simulink model "tank_reactor_no_error_dyn"  (R2020a)
settings: Solver=FixedStepAuto  StartTime=0.0  StopTime=options.T_train  FixedStep=options.dt  RelTol=1e-3
PreLoadFcn:
  | load PIDGainSchedExample.mat
model workspace (MAT data in the model file):
  op_snapshot1 : handle (value not decoded)
undefined symbols (not defined in the file or in its folder): C, Controllers, D, I, N, options, P, sigbuilder_block
libraries: neural x132, simulink x2, simulink_need_slupdate x1
(part 2 of 6)

== system tank_reactor_no_error_dyn/NN/Layer 1/Delays 1 ==
  "p{1}" : Inport  PortDimensions=8
      mask Display: e = 0.06;c1 = [120 230 180]/255;c2 = ([120 230 180]+0)/(256+128);c3 = ([120 230 180]+128)/(256+128);patch([0 1 1 0],[0 0 1 1],c1);patch([0 1 1 1-e 1-e 0+e],[0 0 1 1-e 0+e 0+e],c2);patch([0 0 1 1-e 0+e 0+e],[0 1 1 1-e 1-e 0+e],c3);plot([0 1 1 0 0],[0 0 1 1 0]);
  mux : Mux  Inputs=1
      mask Display: e = 0.06;c1 = [120 150 230]/255;c2 = ([120 150 230]+0)/383;c3 = ([120 150 230]+128)/383;patch([0 1 1 0],[0 0 1 1],c1);patch([0 1 1 1-e 1-e 0+e],[0 0 1 1-e 0+e 0+e],c2);patch([0 0 1 1-e 0+e 0+e],[0 1 1 1-e 1-e 0+e],c3);plot([0 1 1 0 0],[0 0 1 1 0]);disp('Mux')
  "pd{1,1}" : Outport
      mask Display: e = 0.06;c1 = [120 230 180]/255;c2 = ([120 230 180]+0)/(256+128);c3 = ([120 230 180]+128)/(256+128);patch([0 1 1 0],[0 0 1 1],c1);patch([0 1 1 1-e 1-e 0+e],[0 0 1 1-e 0+e 0+e],c2);patch([0 0 1 1-e 0+e 0+e],[0 1 1 1-e 1-e 0+e],c3);plot([0 1 1 0 0],[0 0 1 1 0]);
  wires:
  "p{1}"/1 -> mux/1
  mux/1 -> "pd{1,1}"/1

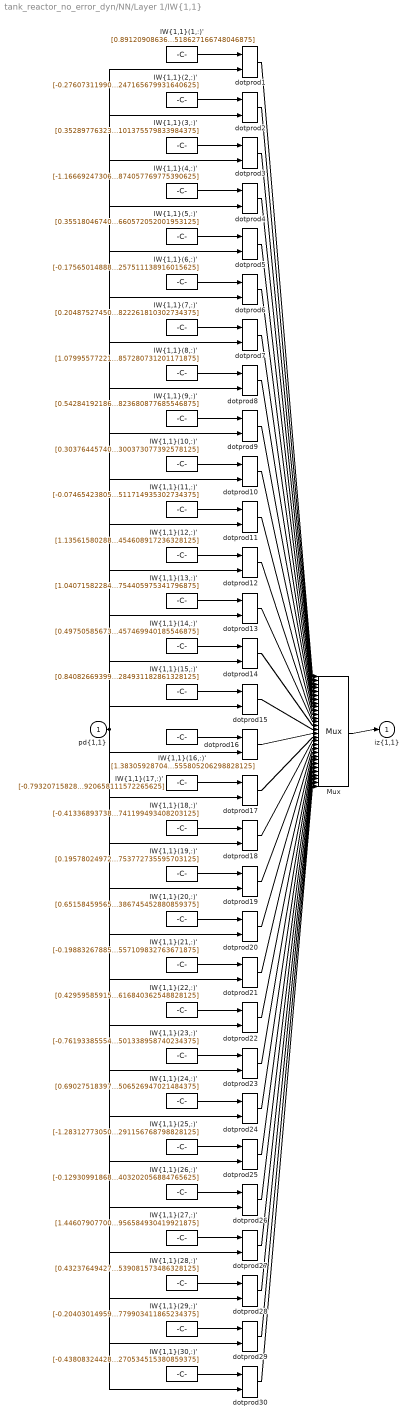
== system tank_reactor_no_error_dyn/NN/Layer 1/IW{1,1} ==
  "pd{1,1}" : Inport  PortDimensions=8
      mask Display: e = 0.06;c1 = [120 230 180]/255;c2 = ([120 230 180]+0)/(256+128);c3 = ([120 230 180]+128)/(256+128);patch([0 1 1 0],[0 0 1 1],c1);patch([0 1 1 1-e 1-e 0+e],[0 0 1 1-e 0+e 0+e],c2);patch([0 0 1 1-e 0+e 0+e],[0 1 1 1-e 1-e 0+e],c3);plot([0 1 1 0 0],[0 0 1 1 0]);
  "IW{1,1}(1,:)'" : Constant  Value=[0.891209086360823743433456911589019000530242919921875;-0.000910908649453586708073793420936681286548264324665069580078125;0.16926229689930305521983200378599576652050018310546875;0.0961010344390704762673749428358860313892364501953125;-0.71802013876261872038497813264257274568080902099609375;-1.2927237305927830046670123920193873345851898193359375;0.90818838200151918993441313432413153350353240966796875;0.427072169502839382726477879259618930518627166748046875]
      mask Display: e = 0.06;c1 = [120 150 230]/255;c2 = ([120 150 230]+0)/383;c3 = ([120 150 230]+128)/383;patch([0 1 1 0],[0 0 1 1],c1);patch([0 1 1 1-e 1-e 0+e],[0 0 1 1-e 0+e 0+e],c2);patch([0 0 1 1-e 0+e 0+e],[0 1 1 1-e 1-e 0+e],c3);plot([0 1 1 0 0],[0 0 1 1 0]);disp('Weights');
  "IW{1,1}(10,:)'" : Constant  Value=[0.303764457407485977125105591767351143062114715576171875;-1.996551308659621160046526711084879934787750244140625;1.2595053737837555996037508521112613379955291748046875;-1.02115406267071673340751658543013036251068115234375;2.473413894732976014978476086980663239955902099609375;-0.7761438730779877115395493092364631593227386474609375;-0.71002775511161775323643041701870970427989959716796875;0.1135875630970302474498367928390507586300373077392578125]
      mask Display: e = 0.06;c1 = [120 150 230]/255;c2 = ([120 150 230]+0)/383;c3 = ([120 150 230]+128)/383;patch([0 1 1 0],[0 0 1 1],c1);patch([0 1 1 1-e 1-e 0+e],[0 0 1 1-e 0+e 0+e],c2);patch([0 0 1 1-e 0+e 0+e],[0 1 1 1-e 1-e 0+e],c3);plot([0 1 1 0 0],[0 0 1 1 0]);disp('Weights');
  "IW{1,1}(11,:)'" : Constant  Value=[-0.07465423805538810853033027115088771097362041473388671875;1.8872792622725416133988574074464850127696990966796875;-0.28367390430513361732067778575583361089229583740234375;-0.60649854229973543251475120996474288403987884521484375;-1.1760495898640888068342746919370256364345550537109375;2.003426546042650802093021411565132439136505126953125;0.51689646511757303404266394863952882587909698486328125;-0.92364179088715070431447884402587078511714935302734375]
      mask Display: e = 0.06;c1 = [120 150 230]/255;c2 = ([120 150 230]+0)/383;c3 = ([120 150 230]+128)/383;patch([0 1 1 0],[0 0 1 1],c1);patch([0 1 1 1-e 1-e 0+e],[0 0 1 1-e 0+e 0+e],c2);patch([0 0 1 1-e 0+e 0+e],[0 1 1 1-e 1-e 0+e],c3);plot([0 1 1 0 0],[0 0 1 1 0]);disp('Weights');
  "IW{1,1}(12,:)'" : Constant  Value=[1.1356158028888374555975815383135341107845306396484375;-0.8606555624373211088595780893228948116302490234375;1.062201621871125656326739772339351475238800048828125;0.385334575489824970873087295331060886383056640625;-1.0206910368916128906136009391047991812229156494140625;-0.76634897790539968642775647822418250143527984619140625;0.71194817031437462873100230353884398937225341796875;-0.684976270533752984448483402957208454608917236328125]
      mask Display: e = 0.06;c1 = [120 150 230]/255;c2 = ([120 150 230]+0)/383;c3 = ([120 150 230]+128)/383;patch([0 1 1 0],[0 0 1 1],c1);patch([0 1 1 1-e 1-e 0+e],[0 0 1 1-e 0+e 0+e],c2);patch([0 0 1 1-e 0+e 0+e],[0 1 1 1-e 1-e 0+e],c3);plot([0 1 1 0 0],[0 0 1 1 0]);disp('Weights');
  "IW{1,1}(13,:)'" : Constant  Value=[1.040715822845224902692962132277898490428924560546875;-1.20594832363064963232091031386516988277435302734375;-0.72554525921453905112912252661772072315216064453125;-0.58377306366834436079926717866328544914722442626953125;0.85741126153984448254874450867646373808383941650390625;-0.71285015732533185683905685436911880970001220703125;-0.294932600157362390103088500836747698485851287841796875;-0.392736442125421081339453621694701723754405975341796875]
      mask Display: e = 0.06;c1 = [120 150 230]/255;c2 = ([120 150 230]+0)/383;c3 = ([120 150 230]+128)/383;patch([0 1 1 0],[0 0 1 1],c1);patch([0 1 1 1-e 1-e 0+e],[0 0 1 1-e 0+e 0+e],c2);patch([0 0 1 1-e 0+e 0+e],[0 1 1 1-e 1-e 0+e],c3);plot([0 1 1 0 0],[0 0 1 1 0]);disp('Weights');
  "IW{1,1}(14,:)'" : Constant  Value=[0.49750585673530112185147800119011662900447845458984375;-0.54863714662622420359383568211342208087444305419921875;0.98098386380823310304322149022482335567474365234375;0.0235222284456758322368497005072640604339540004730224609375;-0.2518678635057340908787182343075983226299285888671875;0.87089778090608327421051626515691168606281280517578125;-0.84448838533145298423931990328128449618816375732421875;0.64158694309444352921190102279069833457469940185546875]
      mask Display: e = 0.06;c1 = [120 150 230]/255;c2 = ([120 150 230]+0)/383;c3 = ([120 150 230]+128)/383;patch([0 1 1 0],[0 0 1 1],c1);patch([0 1 1 1-e 1-e 0+e],[0 0 1 1-e 0+e 0+e],c2);patch([0 0 1 1-e 0+e 0+e],[0 1 1 1-e 1-e 0+e],c3);plot([0 1 1 0 0],[0 0 1 1 0]);disp('Weights');
  "IW{1,1}(15,:)'" : Constant  Value=[0.8408266939989401667077117963344790041446685791015625;-0.6803304612663236827785340210539288818836212158203125;0.909265244574289255297117051668465137481689453125;-1.9435766040642281637929045245982706546783447265625;-0.57838745834684257562940956631791777908802032470703125;0.339153364989726535672076579430722631514072418212890625;0.66688594346699681114642999091302044689655303955078125;-0.98381930870071443440139091762830503284931182861328125]
      mask Display: e = 0.06;c1 = [120 150 230]/255;c2 = ([120 150 230]+0)/383;c3 = ([120 150 230]+128)/383;patch([0 1 1 0],[0 0 1 1],c1);patch([0 1 1 1-e 1-e 0+e],[0 0 1 1-e 0+e 0+e],c2);patch([0 0 1 1-e 0+e 0+e],[0 1 1 1-e 1-e 0+e],c3);plot([0 1 1 0 0],[0 0 1 1 0]);disp('Weights');
  "IW{1,1}(16,:)'" : Constant  Value=[1.3830592870458413568002242755028419196605682373046875;1.0887774896799757851084677895414642989635467529296875;1.271992703112938105647344855242408812046051025390625;-1.1783294637027565965325948127429001033306121826171875;1.1046083450996917463271529413759708404541015625;-0.313172955783324102885245565630611963570117950439453125;-0.708707743855683691691638159682042896747589111328125;0.18575113039401813797013574003358371555805206298828125]
      mask Display: e = 0.06;c1 = [120 150 230]/255;c2 = ([120 150 230]+0)/383;c3 = ([120 150 230]+128)/383;patch([0 1 1 0],[0 0 1 1],c1);patch([0 1 1 1-e 1-e 0+e],[0 0 1 1-e 0+e 0+e],c2);patch([0 0 1 1-e 0+e 0+e],[0 1 1 1-e 1-e 0+e],c3);plot([0 1 1 0 0],[0 0 1 1 0]);disp('Weights');
  "IW{1,1}(17,:)'" : Constant  Value=[-0.7932071582841186963008794919005595147609710693359375;-0.69262888914015141583746526521281339228153228759765625;1.1347110976433001372498665659804828464984893798828125;0.471156780921254736416159403233905322849750518798828125;1.391933236785583449801606548135168850421905517578125;0.76600648986104047377665438034455291926860809326171875;1.4849938450647390819625570657080970704555511474609375;-0.12300708250844562263726089668125496245920658111572265625]
      mask Display: e = 0.06;c1 = [120 150 230]/255;c2 = ([120 150 230]+0)/383;c3 = ([120 150 230]+128)/383;patch([0 1 1 0],[0 0 1 1],c1);patch([0 1 1 1-e 1-e 0+e],[0 0 1 1-e 0+e 0+e],c2);patch([0 0 1 1-e 0+e 0+e],[0 1 1 1-e 1-e 0+e],c3);plot([0 1 1 0 0],[0 0 1 1 0]);disp('Weights');
  "IW{1,1}(18,:)'" : Constant  Value=[-0.41336893738068003489871671263244934380054473876953125;0.34606769462915309976125399771262891590595245361328125;0.6930097657111240483374103860114701092243194580078125;-0.0245843145830253462236214545555412769317626953125;0.0774614107242942162567800323813571594655513763427734375;-1.420788434284315115974095533601939678192138671875;0.7440334973332751733465784127474762499332427978515625;-0.67774743533416892393717034792643971741199493408203125]
      mask Display: e = 0.06;c1 = [120 150 230]/255;c2 = ([120 150 230]+0)/383;c3 = ([120 150 230]+128)/383;patch([0 1 1 0],[0 0 1 1],c1);patch([0 1 1 1-e 1-e 0+e],[0 0 1 1-e 0+e 0+e],c2);patch([0 0 1 1-e 0+e 0+e],[0 1 1 1-e 1-e 0+e],c3);plot([0 1 1 0 0],[0 0 1 1 0]);disp('Weights');
  "IW{1,1}(19,:)'" : Constant  Value=[0.195780249723398913630489914794452488422393798828125;1.5706960428444365351907663352903909981250762939453125;-0.022910753267789296661050002512638457119464874267578125;0.07656576370324440217185468782190582714974880218505859375;-1.8746061388155847993175484589301049709320068359375;1.197653751465737936854338840930722653865814208984375;1.678192708089004003824129540589638054370880126953125;-0.257162313468550618456021084057283587753772735595703125]
      mask Display: e = 0.06;c1 = [120 150 230]/255;c2 = ([120 150 230]+0)/383;c3 = ([120 150 230]+128)/383;patch([0 1 1 0],[0 0 1 1],c1);patch([0 1 1 1-e 1-e 0+e],[0 0 1 1-e 0+e 0+e],c2);patch([0 0 1 1-e 0+e 0+e],[0 1 1 1-e 1-e 0+e],c3);plot([0 1 1 0 0],[0 0 1 1 0]);disp('Weights');
  "IW{1,1}(2,:)'" : Constant  Value=[-0.27607311990221428121827784707420505583286285400390625;3.19576707068835474956358666531741619110107421875;-1.0428488373978215264514801674522459506988525390625;0.33427289240207846976460359655902720987796783447265625;-0.786125397896479061188301784568466246128082275390625;-0.062361390428662490104105842192439013160765171051025390625;1.2065016053652370953130912312190048396587371826171875;-0.394134012811458378511275668643065728247165679931640625]
      mask Display: e = 0.06;c1 = [120 150 230]/255;c2 = ([120 150 230]+0)/383;c3 = ([120 150 230]+128)/383;patch([0 1 1 0],[0 0 1 1],c1);patch([0 1 1 1-e 1-e 0+e],[0 0 1 1-e 0+e 0+e],c2);patch([0 0 1 1-e 0+e 0+e],[0 1 1 1-e 1-e 0+e],c3);plot([0 1 1 0 0],[0 0 1 1 0]);disp('Weights');
  "IW{1,1}(20,:)'" : Constant  Value=[0.65158459565695447945898877151194028556346893310546875;-0.54696539429589241532170262871659360826015472412109375;-0.54826498940842782747751016358961351215839385986328125;-0.65072656451431776236660198264871723949909210205078125;0.0708601621656460844977942770128720439970493316650390625;-1.6283005755519279755816342003527097404003143310546875;0.77614797039212113372030898972298018634319305419921875;1.307748898949637972322079804143868386745452880859375]
      mask Display: e = 0.06;c1 = [120 150 230]/255;c2 = ([120 150 230]+0)/383;c3 = ([120 150 230]+128)/383;patch([0 1 1 0],[0 0 1 1],c1);patch([0 1 1 1-e 1-e 0+e],[0 0 1 1-e 0+e 0+e],c2);patch([0 0 1 1-e 0+e 0+e],[0 1 1 1-e 1-e 0+e],c3);plot([0 1 1 0 0],[0 0 1 1 0]);disp('Weights');
  "IW{1,1}(21,:)'" : Constant  Value=[-0.198832678858577527325479650244233198463916778564453125;-1.5667262584966288319066052281414158642292022705078125;0.60294794988579614170021159225143492221832275390625;1.0351174578473163467862150355358608067035675048828125;0.57511724013551501766272622262476943433284759521484375;-1.9983892082063359207921848792466334998607635498046875;1.087121479066192275553248691721819341182708740234375;-0.085864453590817901851295346205006353557109832763671875]
      mask Display: e = 0.06;c1 = [120 150 230]/255;c2 = ([120 150 230]+0)/383;c3 = ([120 150 230]+128)/383;patch([0 1 1 0],[0 0 1 1],c1);patch([0 1 1 1-e 1-e 0+e],[0 0 1 1-e 0+e 0+e],c2);patch([0 0 1 1-e 0+e 0+e],[0 1 1 1-e 1-e 0+e],c3);plot([0 1 1 0 0],[0 0 1 1 0]);disp('Weights');
  "IW{1,1}(22,:)'" : Constant  Value=[0.42959585915928055754875458660535514354705810546875;1.608771338683758767018616708810441195964813232421875;-1.0989417017832732170745657640509307384490966796875;0.371220710965206202036625882101361639797687530517578125;-0.2473361319530964774759951296800863929092884063720703125;-0.69784269808488785802325082840980030596256256103515625;-0.27799942923109954850957592498161830008029937744140625;0.43439637348526460858266773357172496616840362548828125]
      mask Display: e = 0.06;c1 = [120 150 230]/255;c2 = ([120 150 230]+0)/383;c3 = ([120 150 230]+128)/383;patch([0 1 1 0],[0 0 1 1],c1);patch([0 1 1 1-e 1-e 0+e],[0 0 1 1-e 0+e 0+e],c2);patch([0 0 1 1-e 0+e 0+e],[0 1 1 1-e 1-e 0+e],c3);plot([0 1 1 0 0],[0 0 1 1 0]);disp('Weights');
  "IW{1,1}(23,:)'" : Constant  Value=[-0.76193385554215853350257248166599310934543609619140625;-1.168991754040985764362403642735444009304046630859375;1.16775652995662237998431010055355727672576904296875;-0.8596786858297369438020041343406774103641510009765625;1.1885630047108375340059183145058341324329376220703125;0.6353358394109431817042832335573621094226837158203125;0.73915724568664809002171978136175312101840972900390625;0.087989459536861269750573910641833208501338958740234375]
      mask Display: e = 0.06;c1 = [120 150 230]/255;c2 = ([120 150 230]+0)/383;c3 = ([120 150 230]+128)/383;patch([0 1 1 0],[0 0 1 1],c1);patch([0 1 1 1-e 1-e 0+e],[0 0 1 1-e 0+e 0+e],c2);patch([0 0 1 1-e 0+e 0+e],[0 1 1 1-e 1-e 0+e],c3);plot([0 1 1 0 0],[0 0 1 1 0]);disp('Weights');
  "IW{1,1}(24,:)'" : Constant  Value=[0.6902751839763094920954245026223361492156982421875;-1.1906714422756998761343538717483170330524444580078125;0.82139232284612184731287243266706354916095733642578125;-1.1361593673824572636732455066521652042865753173828125;-0.09408198905645491494365018070311634801328182220458984375;0.379573069658633299727767962394864298403263092041015625;-0.2275798022518404628566912606402183882892131805419921875;0.76388497817848433069087832336663268506526947021484375]
      mask Display: e = 0.06;c1 = [120 150 230]/255;c2 = ([120 150 230]+0)/383;c3 = ([120 150 230]+128)/383;patch([0 1 1 0],[0 0 1 1],c1);patch([0 1 1 1-e 1-e 0+e],[0 0 1 1-e 0+e 0+e],c2);patch([0 0 1 1-e 0+e 0+e],[0 1 1 1-e 1-e 0+e],c3);plot([0 1 1 0 0],[0 0 1 1 0]);disp('Weights');
  "IW{1,1}(25,:)'" : Constant  Value=[-1.283127730500394303447819766006432473659515380859375;-0.82493970737477162469275526746059767901897430419921875;-0.324102141434564117172811847922275774180889129638671875;-0.28127820987730556279160509802750311791896820068359375;-1.0514780139675818926292549804202280938625335693359375;0.7115020200138741923723273430368863046169281005859375;-0.427400400411290071200909324034000746905803680419921875;0.75331051910044621866546776800532825291156768798828125]
      mask Display: e = 0.06;c1 = [120 150 230]/255;c2 = ([120 150 230]+0)/383;c3 = ([120 150 230]+128)/383;patch([0 1 1 0],[0 0 1 1],c1);patch([0 1 1 1-e 1-e 0+e],[0 0 1 1-e 0+e 0+e],c2);patch([0 0 1 1-e 0+e 0+e],[0 1 1 1-e 1-e 0+e],c3);plot([0 1 1 0 0],[0 0 1 1 0]);disp('Weights');
  "IW{1,1}(26,:)'" : Constant  Value=[-0.1293099186855697357856342932791449129581451416015625;2.312536055211477314941248550894670188426971435546875;-1.886850622227131513142239782609976828098297119140625;0.6923975867468554756811727202148176729679107666015625;-0.51896714360574291990957362941117025911808013916015625;-1.232082621271291866804631354170851409435272216796875;0.338074964824850721090143679248285479843616485595703125;-0.17734705034791053979148500729934312403202056884765625]
      mask Display: e = 0.06;c1 = [120 150 230]/255;c2 = ([120 150 230]+0)/383;c3 = ([120 150 230]+128)/383;patch([0 1 1 0],[0 0 1 1],c1);patch([0 1 1 1-e 1-e 0+e],[0 0 1 1-e 0+e 0+e],c2);patch([0 0 1 1-e 0+e 0+e],[0 1 1 1-e 1-e 0+e],c3);plot([0 1 1 0 0],[0 0 1 1 0]);disp('Weights');
  "IW{1,1}(27,:)'" : Constant  Value=[1.4460790770033928875903939115232788026332855224609375;-1.174753989253496389011388600920327007770538330078125;-0.903663094360668051052698501734994351863861083984375;1.2089315703201017893064772579236887395381927490234375;-1.5344822755058282748308329246356151998043060302734375;-1.2575764011052263935397377281333319842815399169921875;0.27661093956695115281263497308827936649322509765625;-0.309828444908113009859107478405348956584930419921875]
      mask Display: e = 0.06;c1 = [120 150 230]/255;c2 = ([120 150 230]+0)/383;c3 = ([120 150 230]+128)/383;patch([0 1 1 0],[0 0 1 1],c1);patch([0 1 1 1-e 1-e 0+e],[0 0 1 1-e 0+e 0+e],c2);patch([0 0 1 1-e 0+e 0+e],[0 1 1 1-e 1-e 0+e],c3);plot([0 1 1 0 0],[0 0 1 1 0]);disp('Weights');
  "IW{1,1}(28,:)'" : Constant  Value=[0.43237649427624680331661011223332025110721588134765625;0.248579972511031643822576597813167609274387359619140625;0.12073941905091711834785428436589427292346954345703125;-0.247775766713915046590699375883559696376323699951171875;-1.41605228232816227063040059874765574932098388671875;-0.250253560258686669204308827829663641750812530517578125;-0.9320172798745807174469746314571239054203033447265625;0.12770737221969341579352885673870332539081573486328125]
      mask Display: e = 0.06;c1 = [120 150 230]/255;c2 = ([120 150 230]+0)/383;c3 = ([120 150 230]+128)/383;patch([0 1 1 0],[0 0 1 1],c1);patch([0 1 1 1-e 1-e 0+e],[0 0 1 1-e 0+e 0+e],c2);patch([0 0 1 1-e 0+e 0+e],[0 1 1 1-e 1-e 0+e],c3);plot([0 1 1 0 0],[0 0 1 1 0]);disp('Weights');
  "IW{1,1}(29,:)'" : Constant  Value=[-0.20403014959684029339115340917487628757953643798828125;-1.2552046966677392614286645766696892678737640380859375;0.422075048629639237862676282020402140915393829345703125;0.457051193739799688220415418982156552374362945556640625;0.813647240052294051793069229461252689361572265625;0.94800113640993155517122659148299135267734527587890625;0.369592747067476079525505383571726270020008087158203125;-1.1506192330556908043348585124476812779903411865234375]
      mask Display: e = 0.06;c1 = [120 150 230]/255;c2 = ([120 150 230]+0)/383;c3 = ([120 150 230]+128)/383;patch([0 1 1 0],[0 0 1 1],c1);patch([0 1 1 1-e 1-e 0+e],[0 0 1 1-e 0+e 0+e],c2);patch([0 0 1 1-e 0+e 0+e],[0 1 1 1-e 1-e 0+e],c3);plot([0 1 1 0 0],[0 0 1 1 0]);disp('Weights');
  "IW{1,1}(3,:)'" : Constant  Value=[0.3528977632348235804471414667204953730106353759765625;0.1308640941319542394527530859704711474478244781494140625;-1.2444579430620941185026140374247916042804718017578125;0.83918272680140393315895153136807493865489959716796875;0.68037558300890565998741976727615110576152801513671875;-0.7022060286452938004941870531183667480945587158203125;-1.100538571020759359697649415466003119945526123046875;-0.6665379620285223349895886713056825101375579833984375]
      mask Display: e = 0.06;c1 = [120 150 230]/255;c2 = ([120 150 230]+0)/383;c3 = ([120 150 230]+128)/383;patch([0 1 1 0],[0 0 1 1],c1);patch([0 1 1 1-e 1-e 0+e],[0 0 1 1-e 0+e 0+e],c2);patch([0 0 1 1-e 0+e 0+e],[0 1 1 1-e 1-e 0+e],c3);plot([0 1 1 0 0],[0 0 1 1 0]);disp('Weights');
  "IW{1,1}(30,:)'" : Constant  Value=[-0.43808324428765110791772485754336230456829071044921875;0.41444371322705408910991309312521480023860931396484375;0.71121513137011527216913009397103451192378997802734375;-0.027277229924096473012706809413430164568126201629638671875;-1.37267882779404803983425154001452028751373291015625;-0.42987169918532674994793296718853525817394256591796875;-1.211486810975065164797115357941947877407073974609375;-0.6761643548908080614268101271591149270534515380859375]
      mask Display: e = 0.06;c1 = [120 150 230]/255;c2 = ([120 150 230]+0)/383;c3 = ([120 150 230]+128)/383;patch([0 1 1 0],[0 0 1 1],c1);patch([0 1 1 1-e 1-e 0+e],[0 0 1 1-e 0+e 0+e],c2);patch([0 0 1 1-e 0+e 0+e],[0 1 1 1-e 1-e 0+e],c3);plot([0 1 1 0 0],[0 0 1 1 0]);disp('Weights');
  "IW{1,1}(4,:)'" : Constant  Value=[-1.16669247306179446610485683777369558811187744140625;1.313151888737838834941840104875154793262481689453125;0.11554526367606703096679865439000423066318035125732421875;0.290758769956429963254862514077103696763515472412109375;-1.21604121550441401922171280602924525737762451171875;-0.34010080794086217093052937343600206077098846435546875;-0.1405823754041759243715858929135720245540142059326171875;0.1962377911275405839575114441686309874057769775390625]
      mask Display: e = 0.06;c1 = [120 150 230]/255;c2 = ([120 150 230]+0)/383;c3 = ([120 150 230]+128)/383;patch([0 1 1 0],[0 0 1 1],c1);patch([0 1 1 1-e 1-e 0+e],[0 0 1 1-e 0+e 0+e],c2);patch([0 0 1 1-e 0+e 0+e],[0 1 1 1-e 1-e 0+e],c3);plot([0 1 1 0 0],[0 0 1 1 0]);disp('Weights');
  "IW{1,1}(5,:)'" : Constant  Value=[0.355180467400776411768248408407089300453662872314453125;-1.1446138133397381064781939130625687539577484130859375;1.2998503170540998130633170148939825594425201416015625;-0.13732972862548187276132694023544900119304656982421875;0.88362338224945358167161657547694630920886993408203125;0.87567478655001151910397538813413120806217193603515625;-0.30563340366142954795947161983349360525608062744140625;-0.33053391115797670085640902470913715660572052001953125]
      mask Display: e = 0.06;c1 = [120 150 230]/255;c2 = ([120 150 230]+0)/383;c3 = ([120 150 230]+128)/383;patch([0 1 1 0],[0 0 1 1],c1);patch([0 1 1 1-e 1-e 0+e],[0 0 1 1-e 0+e 0+e],c2);patch([0 0 1 1-e 0+e 0+e],[0 1 1 1-e 1-e 0+e],c3);plot([0 1 1 0 0],[0 0 1 1 0]);disp('Weights');
  "IW{1,1}(6,:)'" : Constant  Value=[-0.1756501488876137939687538391808629967272281646728515625;1.4205293258788682653204205053043551743030548095703125;-0.300940034305634929179262826437479816377162933349609375;-0.1907224346195115216584525796861271373927593231201171875;-0.9385913103776528654265121076605282723903656005859375;-0.982602586260352683922292271745391190052032470703125;0.523715138108350242163169241393916308879852294921875;-0.447275069227227872747931769481510855257511138916015625]
      mask Display: e = 0.06;c1 = [120 150 230]/255;c2 = ([120 150 230]+0)/383;c3 = ([120 150 230]+128)/383;patch([0 1 1 0],[0 0 1 1],c1);patch([0 1 1 1-e 1-e 0+e],[0 0 1 1-e 0+e 0+e],c2);patch([0 0 1 1-e 0+e 0+e],[0 1 1 1-e 1-e 0+e],c3);plot([0 1 1 0 0],[0 0 1 1 0]);disp('Weights');
  "IW{1,1}(7,:)'" : Constant  Value=[0.2048752745045113454747109926756820641458034515380859375;1.3468461456425815381265920223086141049861907958984375;0.0036662755142019376290718479793895312468521296977996826171875;-0.5200031024826061720744974081753753125667572021484375;-1.6760754682220049271990092165651731193065643310546875;0.57178614216200951414492692492785863578319549560546875;0.7277091077803354846054162408108823001384735107421875;0.1111911977520590733004013372919871471822261810302734375]
      mask Display: e = 0.06;c1 = [120 150 230]/255;c2 = ([120 150 230]+0)/383;c3 = ([120 150 230]+128)/383;patch([0 1 1 0],[0 0 1 1],c1);patch([0 1 1 1-e 1-e 0+e],[0 0 1 1-e 0+e 0+e],c2);patch([0 0 1 1-e 0+e 0+e],[0 1 1 1-e 1-e 0+e],c3);plot([0 1 1 0 0],[0 0 1 1 0]);disp('Weights');
  "IW{1,1}(8,:)'" : Constant  Value=[1.0799557722149959460011814371682703495025634765625;-0.584193546292407717146488721482455730438232421875;-0.419015090910249465849801708827726542949676513671875;0.455745228535148483306471689502359367907047271728515625;-0.97753771333968086931776042547426186501979827880859375;0.475936941338956975844354246873990632593631744384765625;0.62248671937497668249505977655644528567790985107421875;-1.2675430185230183166567030639271251857280731201171875]
      mask Display: e = 0.06;c1 = [120 150 230]/255;c2 = ([120 150 230]+0)/383;c3 = ([120 150 230]+128)/383;patch([0 1 1 0],[0 0 1 1],c1);patch([0 1 1 1-e 1-e 0+e],[0 0 1 1-e 0+e 0+e],c2);patch([0 0 1 1-e 0+e 0+e],[0 1 1 1-e 1-e 0+e],c3);plot([0 1 1 0 0],[0 0 1 1 0]);disp('Weights');
  "IW{1,1}(9,:)'" : Constant  Value=[0.542841921864108289952355335117317736148834228515625;-0.1945527859190485653329005799605511128902435302734375;1.20168877294610343398062468622811138629913330078125;-0.76887048434665572482771267459611408412456512451171875;0.1825073833705465886634300431978772394359111785888671875;-0.42007816328332847621851442454499192535877227783203125;-0.66341656840415763607410326585522852838039398193359375;0.0441394868904689541277974740296485833823680877685546875]
      mask Display: e = 0.06;c1 = [120 150 230]/255;c2 = ([120 150 230]+0)/383;c3 = ([120 150 230]+128)/383;patch([0 1 1 0],[0 0 1 1],c1);patch([0 1 1 1-e 1-e 0+e],[0 0 1 1-e 0+e 0+e],c2);patch([0 0 1 1-e 0+e 0+e],[0 1 1 1-e 1-e 0+e],c3);plot([0 1 1 0 0],[0 0 1 1 0]);disp('Weights');
  Mux : Mux  Inputs=30
      mask Display: e = 0.06;c1 = [120 150 230]/255;c2 = ([120 150 230]+0)/383;c3 = ([120 150 230]+128)/383;patch([0 1 1 0],[0 0 1 1],c1);patch([0 1 1 1-e 1-e 0+e],[0 0 1 1-e 0+e 0+e],c2);patch([0 0 1 1-e 0+e 0+e],[0 1 1 1-e 1-e 0+e],c3);plot([0 1 1 0 0],[0 0 1 1 0]);disp('Mux');
  dotprod{1..30} (30 alike) : neural/Weight Functions/dotprod
  "iz{1,1}" : Outport
      mask Display: e = 0.06;c1 = [120 230 180]/255;c2 = ([120 230 180]+0)/(256+128);c3 = ([120 230 180]+128)/(256+128);patch([0 1 1 0],[0 0 1 1],c1);patch([0 1 1 1-e 1-e 0+e],[0 0 1 1-e 0+e 0+e],c2);patch([0 0 1 1-e 0+e 0+e],[0 1 1 1-e 1-e 0+e],c3);plot([0 1 1 0 0],[0 0 1 1 0]);
  wires:
  "IW{1,1}(1,:)'"/1 -> dotprod1/1
  "pd{1,1}"/1 -> dotprod1/2, dotprod2/2, dotprod3/2, dotprod4/2, dotprod5/2, dotprod6/2, dotprod7/2, dotprod8/2, dotprod9/2, dotprod10/2, dotprod11/2, dotprod12/2, dotprod13/2, dotprod14/2, dotprod15/2, dotprod16/2, dotprod17/2, dotprod18/2, dotprod19/2, dotprod20/2, dotprod21/2, dotprod22/2, dotprod23/2, dotprod24/2, dotprod25/2, dotprod26/2, dotprod27/2, dotprod28/2, dotprod29/2, dotprod30/2
  dotprod1/1 -> Mux/1
  "IW{1,1}(2,:)'"/1 -> dotprod2/1
  dotprod2/1 -> Mux/2
  "IW{1,1}(3,:)'"/1 -> dotprod3/1
  dotprod3/1 -> Mux/3
  "IW{1,1}(4,:)'"/1 -> dotprod4/1
  dotprod4/1 -> Mux/4
  "IW{1,1}(5,:)'"/1 -> dotprod5/1
  dotprod5/1 -> Mux/5
  "IW{1,1}(6,:)'"/1 -> dotprod6/1
  dotprod6/1 -> Mux/6
  "IW{1,1}(7,:)'"/1 -> dotprod7/1
  dotprod7/1 -> Mux/7
  "IW{1,1}(8,:)'"/1 -> dotprod8/1
  dotprod8/1 -> Mux/8
  "IW{1,1}(9,:)'"/1 -> dotprod9/1
  dotprod9/1 -> Mux/9
  "IW{1,1}(10,:)'"/1 -> dotprod10/1
  dotprod10/1 -> Mux/10
  "IW{1,1}(11,:)'"/1 -> dotprod11/1
  dotprod11/1 -> Mux/11
  "IW{1,1}(12,:)'"/1 -> dotprod12/1
  dotprod12/1 -> Mux/12
  "IW{1,1}(13,:)'"/1 -> dotprod13/1
  dotprod13/1 -> Mux/13
  "IW{1,1}(14,:)'"/1 -> dotprod14/1
  dotprod14/1 -> Mux/14
  "IW{1,1}(15,:)'"/1 -> dotprod15/1
  dotprod15/1 -> Mux/15
  "IW{1,1}(16,:)'"/1 -> dotprod16/1
  dotprod16/1 -> Mux/16
  "IW{1,1}(17,:)'"/1 -> dotprod17/1
  dotprod17/1 -> Mux/17
  "IW{1,1}(18,:)'"/1 -> dotprod18/1
  dotprod18/1 -> Mux/18
  "IW{1,1}(19,:)'"/1 -> dotprod19/1
  dotprod19/1 -> Mux/19
  "IW{1,1}(20,:)'"/1 -> dotprod20/1
  dotprod20/1 -> Mux/20
  "IW{1,1}(21,:)'"/1 -> dotprod21/1
  dotprod21/1 -> Mux/21
  "IW{1,1}(22,:)'"/1 -> dotprod22/1
  dotprod22/1 -> Mux/22
  "IW{1,1}(23,:)'"/1 -> dotprod23/1
  dotprod23/1 -> Mux/23
  "IW{1,1}(24,:)'"/1 -> dotprod24/1
  dotprod24/1 -> Mux/24
  "IW{1,1}(25,:)'"/1 -> dotprod25/1
  dotprod25/1 -> Mux/25
  "IW{1,1}(26,:)'"/1 -> dotprod26/1
  dotprod26/1 -> Mux/26
  "IW{1,1}(27,:)'"/1 -> dotprod27/1
  dotprod27/1 -> Mux/27
  "IW{1,1}(28,:)'"/1 -> dotprod28/1
  dotprod28/1 -> Mux/28
  "IW{1,1}(29,:)'"/1 -> dotprod29/1
  dotprod29/1 -> Mux/29
  "IW{1,1}(30,:)'"/1 -> dotprod30/1
  dotprod30/1 -> Mux/30
  Mux/1 -> "iz{1,1}"/1

== system tank_reactor_no_error_dyn/NN/Layer 2/Delays 1 ==
  "p{2}" : Inport  PortDimensions=30
      mask Display: e = 0.06;c1 = [120 230 180]/255;c2 = ([120 230 180]+0)/(256+128);c3 = ([120 230 180]+128)/(256+128);patch([0 1 1 0],[0 0 1 1],c1);patch([0 1 1 1-e 1-e 0+e],[0 0 1 1-e 0+e 0+e],c2);patch([0 0 1 1-e 0+e 0+e],[0 1 1 1-e 1-e 0+e],c3);plot([0 1 1 0 0],[0 0 1 1 0]);
  mux : Mux  Inputs=1
      mask Display: e = 0.06;c1 = [120 150 230]/255;c2 = ([120 150 230]+0)/383;c3 = ([120 150 230]+128)/383;patch([0 1 1 0],[0 0 1 1],c1);patch([0 1 1 1-e 1-e 0+e],[0 0 1 1-e 0+e 0+e],c2);patch([0 0 1 1-e 0+e 0+e],[0 1 1 1-e 1-e 0+e],c3);plot([0 1 1 0 0],[0 0 1 1 0]);disp('Mux')
  "pd{2,1}" : Outport
      mask Display: e = 0.06;c1 = [120 230 180]/255;c2 = ([120 230 180]+0)/(256+128);c3 = ([120 230 180]+128)/(256+128);patch([0 1 1 0],[0 0 1 1],c1);patch([0 1 1 1-e 1-e 0+e],[0 0 1 1-e 0+e 0+e],c2);patch([0 0 1 1-e 0+e 0+e],[0 1 1 1-e 1-e 0+e],c3);plot([0 1 1 0 0],[0 0 1 1 0]);
  wires:
  "p{2}"/1 -> mux/1
  mux/1 -> "pd{2,1}"/1
